simulink model "inverted_pendulum"  (R2024a)
settings: Solver=ode1  StartTime=0.0  StopTime=10.0  FixedStep=0.001  RelTol=1e-3
undefined symbols (not defined in the file): a, b, d, K, lambda, phi
settings Model: Creator=Lenovo  LastModifiedBy=Lenovo

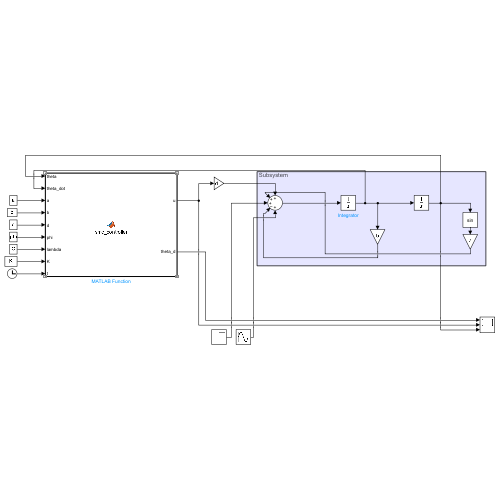
[thumbnail: Simulink's stored preview of the top-level diagram]
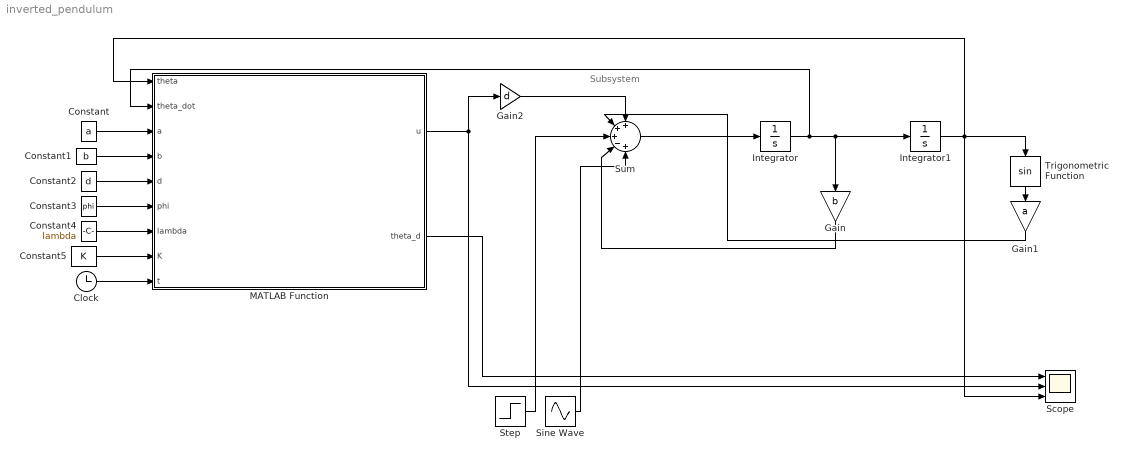
== system inverted_pendulum ==
  note: Subsystem
  Clock : Clock
  Constant : Constant  Value=a
  Constant1 : Constant  Value=b
  Constant2 : Constant  Value=d
  Constant3 : Constant  Value=phi
  Constant4 : Constant  Value=lambda
  Constant5 : Constant  Value=K
  Gain : Gain  Gain=b
  Gain1 : Gain  Gain=a
  Gain2 : Gain  Gain=d
  Integrator : Integrator
  Integrator1 : Integrator
  MATLAB Function : MATLAB Function  TreatAsAtomicUnit=on
  Scope : Scope  NumInputPorts=3
  Sine Wave : Sin  Amplitude=10  Frequency=2  SampleTime=0
  Step : Step  Time=5  After=15  SampleTime=0
  Sum : Sum  Inputs=+++-+
  Trigonometric Function : Trigonometry
  wires:
  Constant/1 -> MATLAB Function/3(a)
  Constant1/1 -> MATLAB Function/4(b)
  Constant2/1 -> MATLAB Function/5(d)
  Constant3/1 -> MATLAB Function/6(phi)
  Constant5/1 -> MATLAB Function/8(K)
  Constant4/1 -> MATLAB Function/7(lambda)
  Clock/1 -> MATLAB Function/9(t)
  MATLAB Function/2(theta_d) -> Scope/1
  MATLAB Function/1(u) -> Scope/2, Gain2/1
  Integrator1/1 -> MATLAB Function/1(theta), Trigonometric Function/1, Scope/3
  Integrator/1 -> Gain/1, Integrator1/1, MATLAB Function/2(theta_dot)
  Sine Wave/1 -> Sum/5
  Step/1 -> Sum/3
  Gain/1 -> Sum/4
  Sum/1 -> Integrator/1
  Gain2/1 -> Sum/1
  Trigonometric Function/1 -> Gain1/1
  Gain1/1 -> Sum/2

== matlab function inverted_pendulum/MATLAB Function ==
  data: theta input; u output; theta_dot input; a input; b input; d input; phi input; lambda input; K input; t input; theta_d output
function  [u,theta_d] = smc_controller(theta, theta_dot, a, b, d, phi, lambda, K, t)
theta_d = 0;
theta_d_dot = 0;
theta_d_dot_dot = 0;
e = theta - theta_d;
e_dot = theta_dot - theta_d_dot;
s = e_dot + lambda*e;
u_eq = (-a*sin(theta)+(b-lambda)*theta_dot)/d;
u_sw = -K*(s/(abs(s)+phi))/d;
%u_sw = -K*sign(s)/d;
u = u_eq + u_sw;
